simulink model "Hydro_With_and_Without_Surge_Tank"  (R2024b)
settings: Solver=ode23t  StartTime=0.0  StopTime=80  RelTol=1e-3
settings Model: Creator=HP  LastModifiedBy=HP

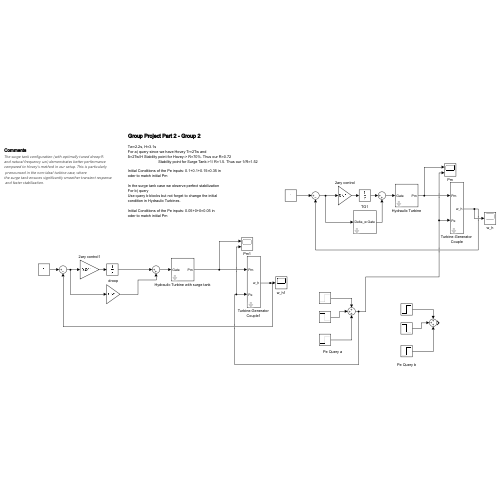
[thumbnail: Simulink's stored preview of the top-level diagram]
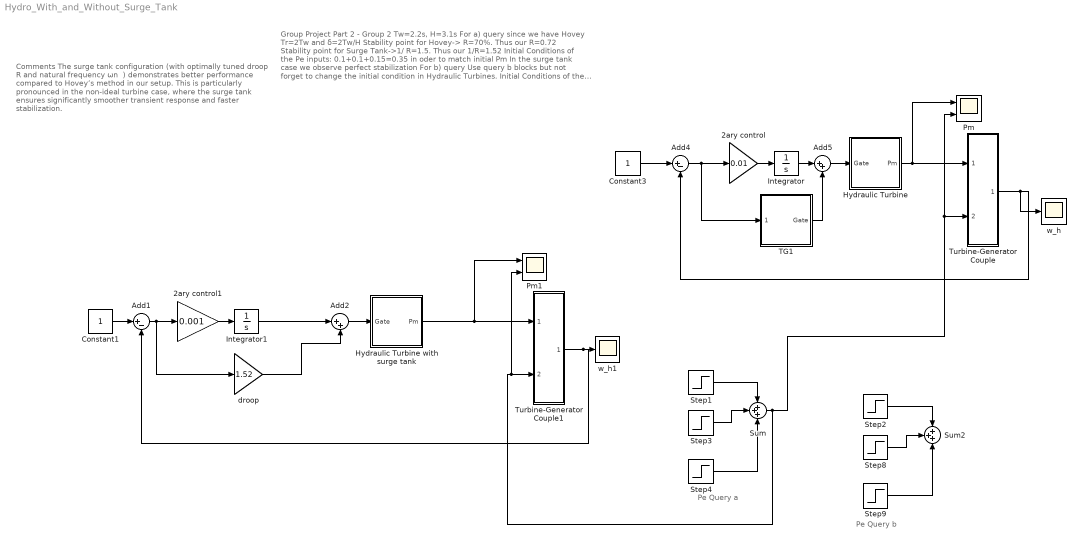
== system Hydro_With_and_Without_Surge_Tank ==
  note: Comments
      | The surge tank configuration (with optimally tuned droop R
      | and natural frequency ωn ​ ) demonstrates better performance
      | compared to Hovey’s method in our setup. This is particularly
      | pronounced in the non-ideal turbine case, where
      | the surge tank ensures significantly smoother transient response
      | and faster stabilization.
  note: Group Project Part 2 - Group 2
      |
      | Tw=2.2s, H=3.1s
      | For a) query since we have Hovey Tr=2Tw and
      | δ=2Tw/H Stability point for Hovey-> R=70%. Thus our R=0.72
      | Stability point for Surge Tank->1/ R=1.5. Thus our 1/R=1.52
      |
      | Initial Conditions of the Pe inputs: 0.1+0.1+0.15=0.35 in
      | oder to match initial Pm
      |
      | In the surge tank case we observe perfect stabilization
      | For b) query
      | Use query b blocks but not forget to change the initial
      | condition in Hydraulic Turbines.
      |
      | Initial Conditions of the Pe inputs: 0.05+0+0=0.05 in
      | oder to match initial Pm
  note: Pe Query a
  note: Pe Query b
  2ary control : Gain  Gain=0.01
  2ary control1 : Gain  Gain=0.001
  Add1 : Sum  Inputs=|+-
  Add2 : Sum  Inputs=|++
  Add4 : Sum  Inputs=|+-
  Add5 : Sum  Inputs=|++
  Constant1 : Constant
  Constant3 : Constant
  Hydraulic Turbine : Subsystem  mask{Tw=2.2, ini=0.35}
      mask prompts: Tw "Water Constant"; ini "Initial Pm"
  Hydraulic Turbine with surge tank : Subsystem  mask{Tw=2.2, ini=0.35, wn=0.01}
      mask prompts: Tw "Water Constant"; ini "Initial Pm"; wn "Natural Frequency"
  Integrator : Integrator  InitialCondition=0.35
  Integrator1 : Integrator  InitialCondition=0.35
  Pm : Scope  NumInputPorts=2
  Pm1 : Scope  NumInputPorts=2
  Step1 : Step  Time=5  Before=0.10  After=0.35  SampleTime=0
  Step2 : Step  Time=5  Before=0.05  After=0.25  SampleTime=0
  Step3 : Step  Time=15  Before=0.10  After=-0.30  SampleTime=0
  Step4 : Step  Time=25  Before=0.15  After=0.45  SampleTime=0
  Step8 : Step  Time=10  After=-0.15  SampleTime=0
  Step9 : Step  Time=15  After=0.1  SampleTime=0
  Sum : Sum  Inputs=+++
  Sum2 : Sum  Inputs=+++
  TG1 : Subsystem  mask{Tr=4*2.2, ini=0, delta=2*2.2/3.1, R=0.72}
      mask prompts: Tr "Transient time"; ini "Initial gate"; delta "Delta Gain"; R "Droop"
  Turbine-Generator Couple : Subsystem  mask{Hh=3.1, w_ini=1}
      mask prompts: Hh "H/E Inertia Constant"; w_ini "Initial omega"
  Turbine-Generator Couple1 : Subsystem  mask{Hh=3.1, w_ini=1}
      mask prompts: Hh "H/E Inertia Constant"; w_ini "Initial omega"
  droop : Gain  Gain=1.52
  w_h : Scope
  w_h1 : Scope
  wires:
  Turbine-Generator Couple/1(w_h) -> Add4/2, w_h/1
  Hydraulic Turbine/1(Pm) -> Pm/1, Turbine-Generator Couple/1(Pm)
  Step1/1 -> Sum/1
  Step3/1 -> Sum/2
  Step4/1 -> Sum/3
  Step2/1 -> Sum2/1
  Step8/1 -> Sum2/2
  Step9/1 -> Sum2/3
  Sum/1 -> Pm1/2, Turbine-Generator Couple1/2(Pe), Turbine-Generator Couple/2(Pe), Pm/2
  Constant3/1 -> Add4/1
  TG1/1(Gate) -> Add5/2
  Add4/1 -> TG1/1(Delta_w), 2ary control/1
  Integrator/1 -> Add5/1
  2ary control/1 -> Integrator/1
  Add5/1 -> Hydraulic Turbine/1(Gate)
  Add1/1 -> droop/1, 2ary control1/1
  Turbine-Generator Couple1/1(w_h) -> Add1/2, w_h1/1
  Integrator1/1 -> Add2/1
  droop/1 -> Add2/2
  Constant1/1 -> Add1/1
  2ary control1/1 -> Integrator1/1
  Add2/1 -> Hydraulic Turbine with surge tank/1(Gate)
  Hydraulic Turbine with surge tank/1(Pm) -> Pm1/1, Turbine-Generator Couple1/1(Pm)

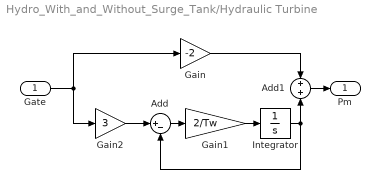
== system Hydro_With_and_Without_Surge_Tank/Hydraulic Turbine ==
  Gate : Inport
  Add : Sum  Inputs=|+-
  Add1 : Sum  Inputs=+|+
  Gain : Gain  Gain=-2
  Gain1 : Gain  Gain=2/Tw
  Gain2 : Gain  Gain=3
  Integrator : Integrator  InitialCondition=3*ini
  Pm : Outport
  wires:
  Add1/1 -> Pm/1
  Integrator/1 -> Add1/2, Add/2
  Gain/1 -> Add1/1
  Gate/1 -> Gain2/1, Gain/1
  Add/1 -> Gain1/1
  Gain1/1 -> Integrator/1
  Gain2/1 -> Add/1

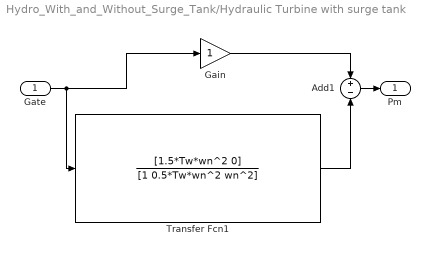
== system Hydro_With_and_Without_Surge_Tank/Hydraulic Turbine with surge tank ==
  Gate : Inport
  Add1 : Sum  Inputs=+|-
  Gain : Gain
  Transfer Fcn1 : TransferFcn  Numerator=[1.5*Tw*wn^2 0]  Denominator=[1 0.5*Tw*wn^2 wn^2]
  Pm : Outport
  wires:
  Gate/1 -> Transfer Fcn1/1, Gain/1
  Gain/1 -> Add1/1
  Add1/1 -> Pm/1
  Transfer Fcn1/1 -> Add1/2

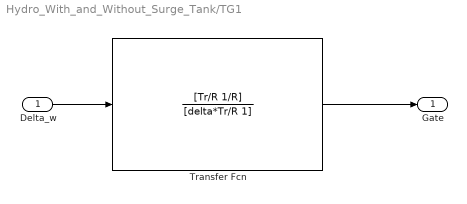
== system Hydro_With_and_Without_Surge_Tank/TG1 ==
  Delta_w : Inport
  Transfer Fcn : TransferFcn  Numerator=[Tr/R 1/R]  Denominator=[delta*Tr/R 1]
  Gate : Outport
  wires:
  Transfer Fcn/1 -> Gate/1
  Delta_w/1 -> Transfer Fcn/1

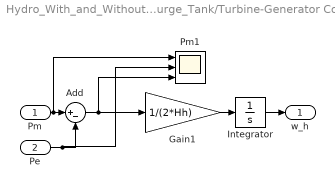
== system Hydro_With_and_Without_Surge_Tank/Turbine-Generator Couple ==
  Pm : Inport
  Pe : Inport  Port=2
  Add : Sum  Inputs=|+-
  Gain1 : Gain  Gain=1/(2*Hh)
  Integrator : Integrator  InitialCondition=w_ini
  Pm1 : Scope  NumInputPorts=3
  w_h : Outport
  wires:
  Pm/1 -> Pm1/1, Add/1
  Gain1/1 -> Integrator/1
  Integrator/1 -> w_h/1
  Pe/1 -> Pm1/2, Add/2
  Add/1 -> Pm1/3, Gain1/1

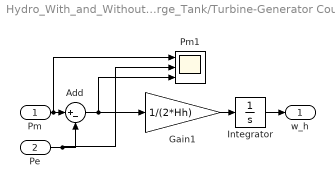
== system Hydro_With_and_Without_Surge_Tank/Turbine-Generator Couple1 ==
  Pm : Inport
  Pe : Inport  Port=2
  Add : Sum  Inputs=|+-
  Gain1 : Gain  Gain=1/(2*Hh)
  Integrator : Integrator  InitialCondition=w_ini
  Pm1 : Scope  NumInputPorts=3
  w_h : Outport
  wires:
  Add/1 -> Gain1/1, Pm1/3
  Pe/1 -> Add/2, Pm1/2
  Integrator/1 -> w_h/1
  Gain1/1 -> Integrator/1
  Pm/1 -> Add/1, Pm1/1
